simulink model "motor_2"  (R2023a)
settings: Solver=ode15s  StartTime=0.0  StopTime=sim_end_time  MaxStep=0.0001  RelTol=1e-3
values from neighbouring files (symbols this model uses):
  alpha_cu = 3.9 *10^-3    (= 0.0039)    [BLDC_Motor_params_03.m]    (also in DC_Motor_params_01.m; DC_Motor_params_02.m; DC_Motor_params_04.m; DC_Motor_params_05.m)
  b_m2 = .01    (= 0.01)    [DC_Motor_params_02.m]
  C_t2 = 66.49    [DC_Motor_params_02.m]
  ENABLE_SATURATIONS = 1    [run_flags.m]
  J_eq2 = J_2 + 1/8 * m_2 * d_2^2 / r_2^2    [DC_Motor_params_02.m]
  K_d2 = 0.07064    [PID_tuning.m]
  k_e2 = 0.56    [DC_Motor_params_02.m]
  K_i2 = 0    [PID_tuning.m]
  K_p2 = 15.5368    [PID_tuning.m]
  k_t2 = 0.56    [DC_Motor_params_02.m]
  L_a2 = 3*10^-3    (= 0.003)    [DC_Motor_params_02.m]
  r_2 = 5    [DC_Motor_params_02.m]
  r_a2_20 = 0.25    [DC_Motor_params_02.m]
  res_term_2 = 3.15    [DC_Motor_params_02.m]
  T_s0_2 = 20    [use_machine_1.m]    (also in use_solo_motor_2.m)
  theta_m0_2 = 0    [use_machine_1.m]    (also in use_solo_motor_2.m = 3.14159265359)
  voltage_2 = 110    [DC_Motor_params_02.m]
settings Model: Creator=Usuario  LastModifiedBy=Usuario

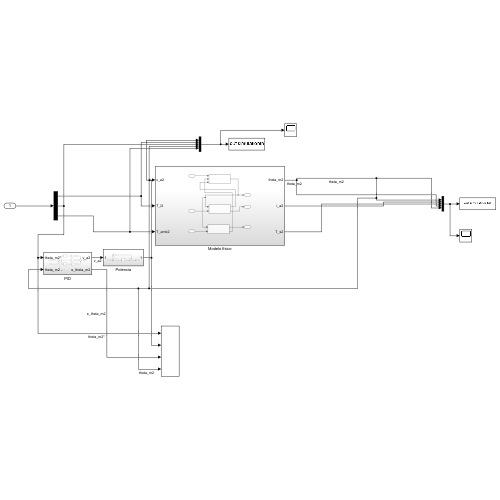
[thumbnail: Simulink's stored preview of the top-level diagram]
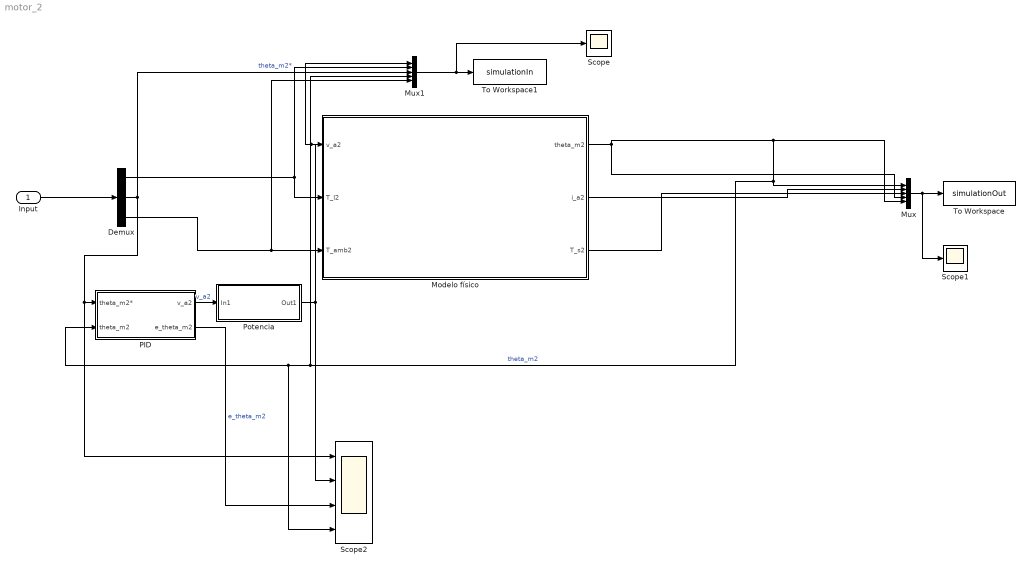
== system motor_2 ==
  Input : Inport
  Demux : Demux  Outputs=3
  Modelo físico : Subsystem
  Mux : Mux  Inputs=5
  Mux1 : Mux  Inputs=5
  PID : Subsystem
  Potencia : Subsystem
  Scope : Scope
  Scope1 : Scope
  Scope2 : Scope  NumInputPorts=4
  To Workspace : ToWorkspace  VariableName=simulationOut  SaveFormat=Timeseries  SampleTime=-1
  To Workspace1 : ToWorkspace  VariableName=simulationIn  SaveFormat=Timeseries  SampleTime=-1
  wires:
  Modelo físico/3(T_s2) -> Mux/3
  Modelo físico/1(theta_m2) -> Mux/5, Mux/1, Mux1/4, PID/2(theta_m2), Scope2/4, Mux/4  "theta_m2"
  PID/2(e_theta_m2) -> Scope2/3  "e_theta_m2"
  PID/1(v_a2) -> Potencia/1(In1)  "v_a2"
  Demux/1 -> Modelo físico/2(T_l2), Mux1/2
  Mux/1 -> Scope1/1, To Workspace/1
  Demux/2 -> Scope2/1, PID/1(theta_m2*), Mux1/3  "theta_m2*"
  Demux/3 -> Mux1/5, Modelo físico/3(T_amb2)
  Modelo físico/2(i_a2) -> Mux/2
  Mux1/1 -> Scope/1, To Workspace1/1
  Input/1 -> Demux/1
  Potencia/1(Out1) -> Mux1/1, Modelo físico/1(v_a2), Scope2/2

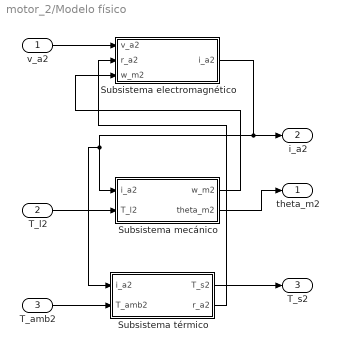
== system motor_2/Modelo físico ==
  v_a2 : Inport
  T_l2 : Inport  Port=2
  T_amb2 : Inport  Port=3
  Subsistema electromagnético : Subsystem
  Subsistema mecánico : Subsystem
  Subsistema térmico : Subsystem
  theta_m2 : Outport
  i_a2 : Outport  Port=2
  T_s2 : Outport  Port=3
  wires:
  Subsistema electromagnético/1(i_a2) -> Subsistema térmico/1(i_a2), Subsistema mecánico/1(i_a2), i_a2/1
  v_a2/1 -> Subsistema electromagnético/1(v_a2)
  T_l2/1 -> Subsistema mecánico/2(T_l2)
  T_amb2/1 -> Subsistema térmico/2(T_amb2)
  Subsistema térmico/1(T_s2) -> T_s2/1
  Subsistema térmico/2(r_a2) -> Subsistema electromagnético/2(r_a2)
  Subsistema mecánico/1(w_m2) -> Subsistema electromagnético/3(w_m2)
  Subsistema mecánico/2(theta_m2) -> theta_m2/1

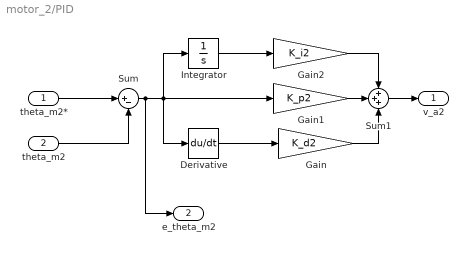
== system motor_2/PID ==
  theta_m2* : Inport
  theta_m2 : Inport  Port=2
  Derivative : Derivative
  Gain : Gain  Gain=K_d2
  Gain1 : Gain  Gain=K_p2
  Gain2 : Gain  Gain=K_i2
  Integrator : Integrator
  Sum : Sum  Inputs=|+-
  Sum1 : Sum  Inputs=+++
  v_a2 : Outport
  e_theta_m2 : Outport  Port=2
  wires:
  theta_m2*/1 -> Sum/1
  theta_m2/1 -> Sum/2
  Sum/1 -> e_theta_m2/1, Integrator/1, Gain1/1, Derivative/1
  Integrator/1 -> Gain2/1
  Derivative/1 -> Gain/1
  Gain1/1 -> Sum1/2
  Gain2/1 -> Sum1/1
  Sum1/1 -> v_a2/1
  Gain/1 -> Sum1/3

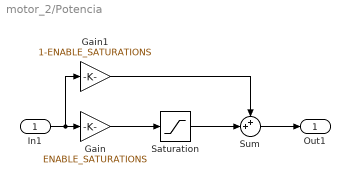
== system motor_2/Potencia ==
  In1 : Inport
  Gain : Gain  Gain=ENABLE_SATURATIONS
  Gain1 : Gain  Gain=1-ENABLE_SATURATIONS
  Saturation : Saturate  UpperLimit=+voltage_2  LowerLimit=-voltage_2
  Sum : Sum  Inputs=++|
  Out1 : Outport
  wires:
  Saturation/1 -> Sum/2
  Gain/1 -> Saturation/1
  In1/1 -> Gain1/1, Gain/1
  Sum/1 -> Out1/1
  Gain1/1 -> Sum/1

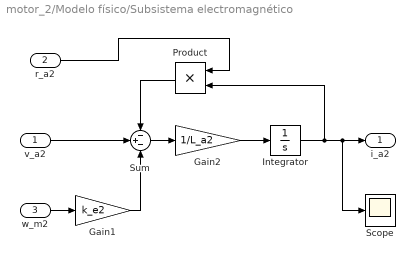
== system motor_2/Modelo físico/Subsistema electromagnético ==
  v_a2 : Inport
  r_a2 : Inport  Port=2
  w_m2 : Inport  Port=3
  Gain1 : Gain  Gain=k_e2
  Gain2 : Gain  Gain=1/L_a2
  Integrator : Integrator
  Product : Product
  Scope : Scope
  Sum : Sum  Inputs=-+-
  i_a2 : Outport
  wires:
  v_a2/1 -> Sum/2
  Integrator/1 -> Product/2, Scope/1, i_a2/1
  Product/1 -> Sum/1
  w_m2/1 -> Gain1/1
  Gain1/1 -> Sum/3
  Sum/1 -> Gain2/1
  Gain2/1 -> Integrator/1
  r_a2/1 -> Product/1

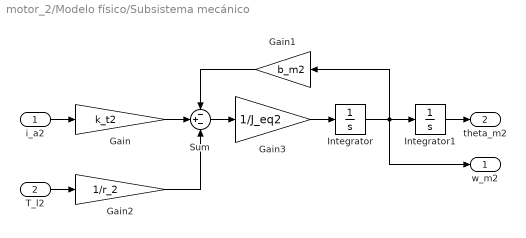
== system motor_2/Modelo físico/Subsistema mecánico ==
  i_a2 : Inport
  T_l2 : Inport  Port=2
  Gain : Gain  Gain=k_t2
  Gain1 : Gain  Gain=b_m2
  Gain2 : Gain  Gain=1/r_2
  Gain3 : Gain  Gain=1/J_eq2
  Integrator : Integrator
  Integrator1 : Integrator  InitialCondition=theta_m0_2
  Sum : Sum  Inputs=-+-
  w_m2 : Outport
  theta_m2 : Outport  Port=2
  wires:
  i_a2/1 -> Gain/1
  Gain/1 -> Sum/2
  Integrator/1 -> w_m2/1, Gain1/1, Integrator1/1
  Gain1/1 -> Sum/1
  T_l2/1 -> Gain2/1
  Gain3/1 -> Integrator/1
  Sum/1 -> Gain3/1
  Integrator1/1 -> theta_m2/1
  Gain2/1 -> Sum/3

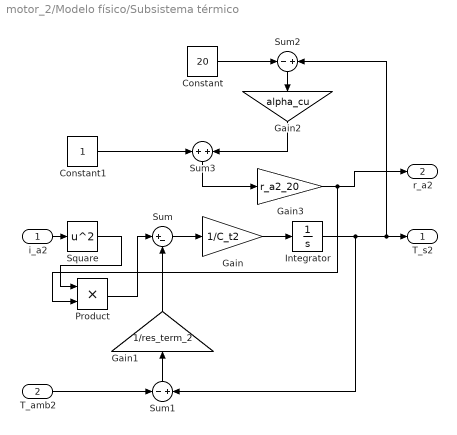
== system motor_2/Modelo físico/Subsistema térmico ==
  i_a2 : Inport
  T_amb2 : Inport  Port=2
  Constant : Constant  Value=20
  Constant1 : Constant
  Gain : Gain  Gain=1/C_t2
  Gain1 : Gain  Gain=1/res_term_2
  Gain2 : Gain  Gain=alpha_cu
  Gain3 : Gain  Gain=r_a2_20
  Integrator : Integrator  InitialCondition=T_s0_2
  Product : Product
  Square : Math  Operator=square
  Sum : Sum  Inputs=|+-
  Sum1 : Sum  Inputs=-|+
  Sum2 : Sum  Inputs=-|+
  Sum3 : Sum  Inputs=+|+
  T_s2 : Outport
  r_a2 : Outport  Port=2
  wires:
  i_a2/1 -> Square/1
  Sum3/1 -> Gain3/1
  Gain2/1 -> Sum3/2
  Square/1 -> Product/1
  Gain3/1 -> Product/2, r_a2/1
  Sum2/1 -> Gain2/1
  T_amb2/1 -> Sum1/1
  Constant1/1 -> Sum3/1
  Gain/1 -> Integrator/1
  Sum/1 -> Gain/1
  Integrator/1 -> Sum1/2, Sum2/2, T_s2/1
  Constant/1 -> Sum2/1
  Sum1/1 -> Gain1/1
  Gain1/1 -> Sum/2
  Product/1 -> Sum/1
